simulink library "StdAnimationLibrary2017"  (R2020a)
settings: Solver=VariableStepAuto  StartTime=0.0  StopTime=10.0  RelTol=1e-3
undefined symbols (not defined in the file): CONST_No_Animation, P_AnimationPeriod, P_CIE_GAMMA, P_CIE_PWM, P_DefaultValue, P_EndValue, P_Nb_Seq_Max, P_SequenceNum_perAnim, P_StartValue, P_TRamp, P_TStart
libraries: simulink x5, $bdroot x1
settings Model: Creator=mchawa  LastModifiedBy=oashraf
settings DataIOCC: ReturnWorkspaceOutputs=off
settings DebuggingCC: ArithmeticOperatorsInVariantConditions=warning
settings SFSimCC: SimUseLocalCustomCode=off  CustomCodeUndefinedFunction=UseInterfaceOnly
settings RTWCC: RTWUseLocalCustomCode=off

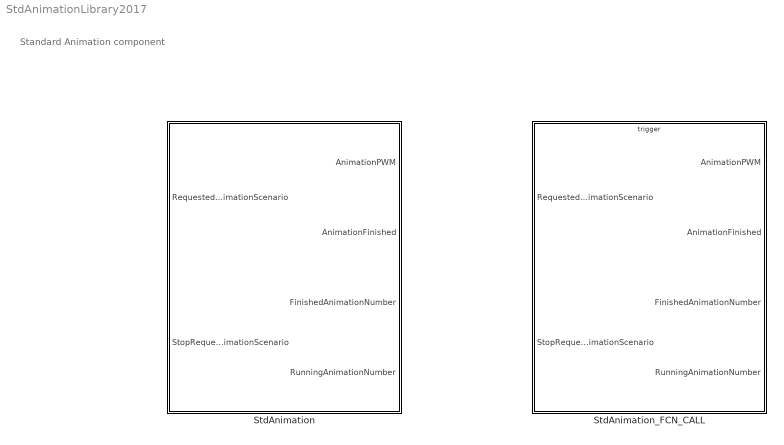
== system StdAnimationLibrary2017 ==
  note: Standard Animation component
  StdAnimation : Subsystem
  StdAnimation_FCN_CALL : Subsystem  TreatAsAtomicUnit=on

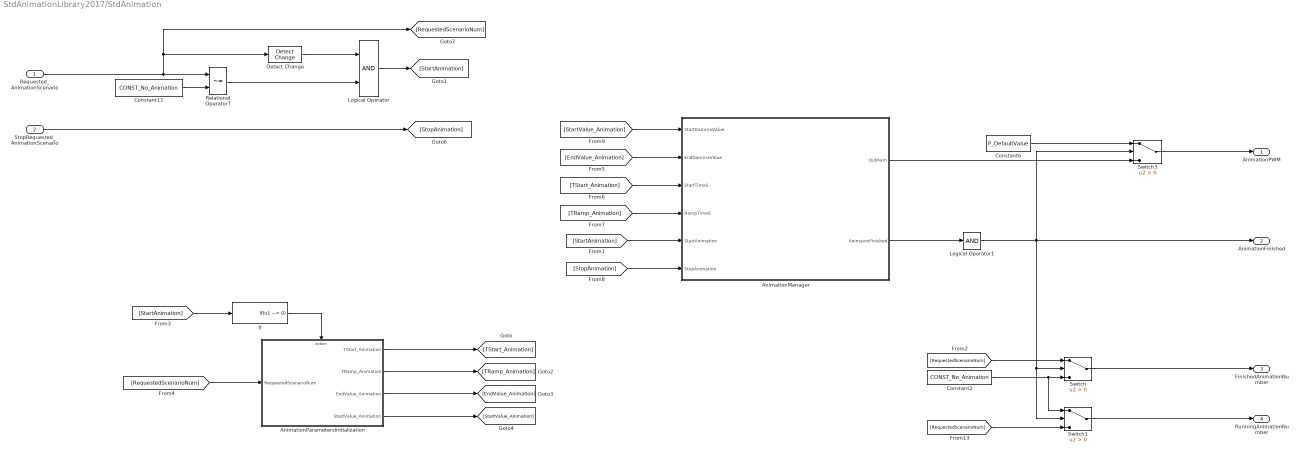
== system StdAnimationLibrary2017/StdAnimation ==
  Requested_AnimationScenario : Inport
  StopRequested_AnimationScenario : Inport  Port=2  PortDimensions=1
  AnimationManager : Subsystem  TreatAsAtomicUnit=on
  AnimationParametersInitialization : Subsystem  TreatAsAtomicUnit=on
  Constant11 : Constant  Value=CONST_No_Animation  OutDataTypeStr=uint8
  Constant2 : Constant  Value=CONST_No_Animation
  Constant6 : Constant  Value=P_DefaultValue
  Detect Change : simulink/Logic and Bit Operations/Detect Change  vinit=0  OutDataTypeStr=boolean
  If : If  IfExpression=u1 ~= 0  ShowElse=off
  Logical Operator : Logic  IconShape=distinctive  AllPortsSameDT=off  OutDataTypeStr=boolean
  Logical Operator1 : Logic  Inputs=1  AllPortsSameDT=off  OutDataTypeStr=boolean
  Relational Operator7 : RelationalOperator  Operator=~=  OutDataTypeStr=boolean  RndMeth=Simplest
  Switch : Switch  Criteria=u2 > Threshold
  Switch1 : Switch  Criteria=u2 > Threshold
  Switch3 : Switch  Criteria=u2 > Threshold
  AnimationPWM : Outport  VectorParamsAs1DForOutWhenUnconnected=off
  AnimationFinished : Outport  Port=2  VectorParamsAs1DForOutWhenUnconnected=off
  FinishedAnimationNumber : Outport  Port=3  VectorParamsAs1DForOutWhenUnconnected=off
  RunningAnimationNumber : Outport  Port=4  VectorParamsAs1DForOutWhenUnconnected=off
  wires:
  AnimationManager/2(AnimaionFinished) -> Logical Operator1/1
  Detect Change/1 -> Logical Operator/1
  AnimationManager/1(OutPwm) -> Switch3/3
  Requested_AnimationScenario/1 -> [RequestedScenarioNum], Detect Change/1, Relational Operator7/1
  [StartAnimation] -> AnimationManager/5(StartAnimation)
  [RequestedScenarioNum] -> Switch1/3
  Logical Operator/1 -> [StartAnimation]
  If/1 -> AnimationParametersInitialization/Action
  [EndValue_Animation] -> AnimationManager/2(EndGammaValue)
  [StartAnimation] -> If/1
  Constant2/1 -> Switch1/1, Switch/3
  [StartValue_Animation] -> AnimationManager/1(StartGammaValue)
  AnimationParametersInitialization/2(TRamp_Animation) -> [TRamp_Animation]
  AnimationParametersInitialization/3(EndValue_Animation) -> [EndValue_Animation]
  [RequestedScenarioNum] -> Switch/1
  Relational Operator7/1 -> Logical Operator/2
  [TStart_Animation] -> AnimationManager/3(StartTimeS)
  [StopAnimation] -> AnimationManager/6(StopAnimation)
  AnimationParametersInitialization/1(TStart_Animation) -> [TStart_Animation]
  [TRamp_Animation] -> AnimationManager/4(RampTimeS)
  Switch1/1 -> RunningAnimationNumber/1
  Switch/1 -> FinishedAnimationNumber/1
  Constant11/1 -> Relational Operator7/2
  StopRequested_AnimationScenario/1 -> [StopAnimation]
  [RequestedScenarioNum] -> AnimationParametersInitialization/1(RequestedScenarioNum)
  Constant6/1 -> Switch3/1
  Switch3/1 -> AnimationPWM/1
  Logical Operator1/1 -> AnimationFinished/1, Switch3/2, Switch/2, Switch1/2
  AnimationParametersInitialization/4(StartValue_Animation) -> [StartValue_Animation]

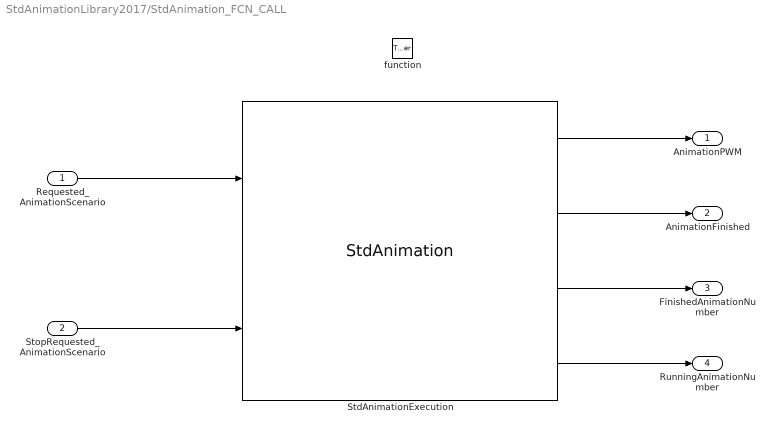
== system StdAnimationLibrary2017/StdAnimation_FCN_CALL ==
  Requested_AnimationScenario : Inport
  StopRequested_AnimationScenario : Inport  Port=2  PortDimensions=1
  function : TriggerPort  TriggerType=function-call  VariantControl=Variant
  StdAnimationExecution : $bdroot/StdAnimation  SystemSampleTime=-1  Latency=0  AutoFrameSizeCalculation=off
      link override AnimationManager/AnimationParametersManager/Detect Change: vinit=P_SequenceNum_perAnim
  AnimationPWM : Outport  VectorParamsAs1DForOutWhenUnconnected=off
  AnimationFinished : Outport  Port=2  VectorParamsAs1DForOutWhenUnconnected=off
  FinishedAnimationNumber : Outport  Port=3  VectorParamsAs1DForOutWhenUnconnected=off
  RunningAnimationNumber : Outport  Port=4  VectorParamsAs1DForOutWhenUnconnected=off
  wires:
  Requested_AnimationScenario/1 -> StdAnimationExecution/1
  StopRequested_AnimationScenario/1 -> StdAnimationExecution/2
  StdAnimationExecution/4 -> RunningAnimationNumber/1
  StdAnimationExecution/3 -> FinishedAnimationNumber/1
  StdAnimationExecution/1 -> AnimationPWM/1
  StdAnimationExecution/2 -> AnimationFinished/1

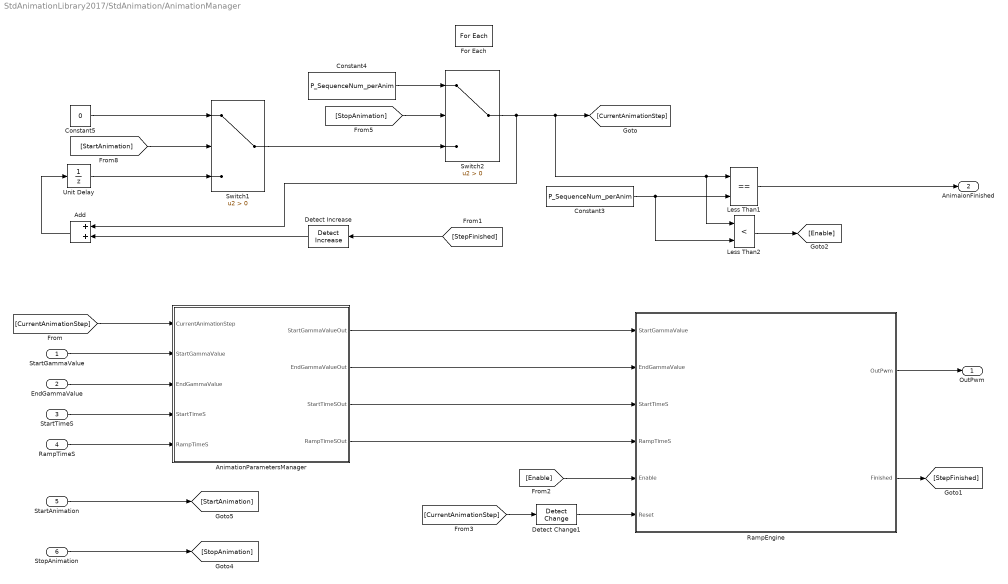
== system StdAnimationLibrary2017/StdAnimation/AnimationManager ==
  StartGammaValue : Inport  Partition=on  PartitionDimension=2  PartitionWidth=1  PartitionOffset=0
  EndGammaValue : Inport  Port=2  Partition=on  PartitionDimension=2  PartitionWidth=1  PartitionOffset=0
  StartTimeS : Inport  Port=3  Partition=on  PartitionDimension=2  PartitionWidth=1  PartitionOffset=0
  RampTimeS : Inport  Port=4  Partition=on  PartitionDimension=2  PartitionWidth=1  PartitionOffset=0
  StartAnimation : Inport  Port=5  OutDataTypeStr=boolean
  StopAnimation : Inport  Port=6  OutDataTypeStr=boolean
  Add : Sum
  AnimationParametersManager : Subsystem  TreatAsAtomicUnit=on
  Constant3 : Constant  Value=P_SequenceNum_perAnim
  Constant4 : Constant  Value=P_SequenceNum_perAnim  OutDataTypeStr=uint8
  Constant5 : Constant  Value=0  OutDataTypeStr=uint8
  Detect Change1 : simulink/Logic and Bit Operations/Detect Change  vinit=0  OutDataTypeStr=boolean
  Detect Increase : simulink/Logic and Bit Operations/Detect Increase  vinit=0.0  OutDataTypeStr=boolean
  For Each : ForEach  DisableCoverage=on
  Less Than1 : RelationalOperator  Operator===  OutDataTypeStr=boolean  RndMeth=Simplest
  Less Than2 : RelationalOperator  Operator=<  OutDataTypeStr=boolean  RndMeth=Simplest
  RampEngine : Subsystem
  Switch1 : Switch  Criteria=u2 > Threshold  OutDataTypeStr=uint8
  Switch2 : Switch  Criteria=u2 > Threshold  OutDataTypeStr=uint8
  Unit Delay : UnitDelay  InitialCondition=P_SequenceNum_perAnim  SampleTime=-1  HasFrameUpgradeWarning=on
  OutPwm : Outport  ConcatenationDimension=1  VectorParamsAs1DForOutWhenUnconnected=off
  AnimaionFinished : Outport  Port=2  ConcatenationDimension=1  VectorParamsAs1DForOutWhenUnconnected=off
  wires:
  [CurrentAnimationStep] -> AnimationParametersManager/1(CurrentAnimationStep)
  Switch1/1 -> Switch2/3
  [CurrentAnimationStep] -> Detect Change1/1
  Constant5/1 -> Switch1/1
  [StartAnimation] -> Switch1/2
  EndGammaValue/1 -> AnimationParametersManager/3(EndGammaValue)
  Unit Delay/1 -> Switch1/3
  Add/1 -> Unit Delay/1
  [Enable] -> RampEngine/5(Enable)
  [StepFinished] -> Detect Increase/1
  Detect Increase/1 -> Add/2
  Constant4/1 -> Switch2/1
  RampEngine/2(Finished) -> [StepFinished]
  [StopAnimation] -> Switch2/2
  AnimationParametersManager/1(StartGammaValueOut) -> RampEngine/1(StartGammaValue)
  AnimationParametersManager/2(EndGammaValueOut) -> RampEngine/2(EndGammaValue)
  StartTimeS/1 -> AnimationParametersManager/4(StartTimeS)
  RampTimeS/1 -> AnimationParametersManager/5(RampTimeS)
  AnimationParametersManager/3(StartTimeSOut) -> RampEngine/3(StartTimeS)
  AnimationParametersManager/4(RampTimeSOut) -> RampEngine/4(RampTimeS)
  StartAnimation/1 -> [StartAnimation]
  StopAnimation/1 -> [StopAnimation]
  Detect Change1/1 -> RampEngine/6(Reset)
  RampEngine/1(OutPwm) -> OutPwm/1
  Constant3/1 -> Less Than1/2, Less Than2/2
  StartGammaValue/1 -> AnimationParametersManager/2(StartGammaValue)
  Switch2/1 -> Less Than2/1, Less Than1/1, [CurrentAnimationStep], Add/1
  Less Than1/1 -> AnimaionFinished/1
  Less Than2/1 -> [Enable]

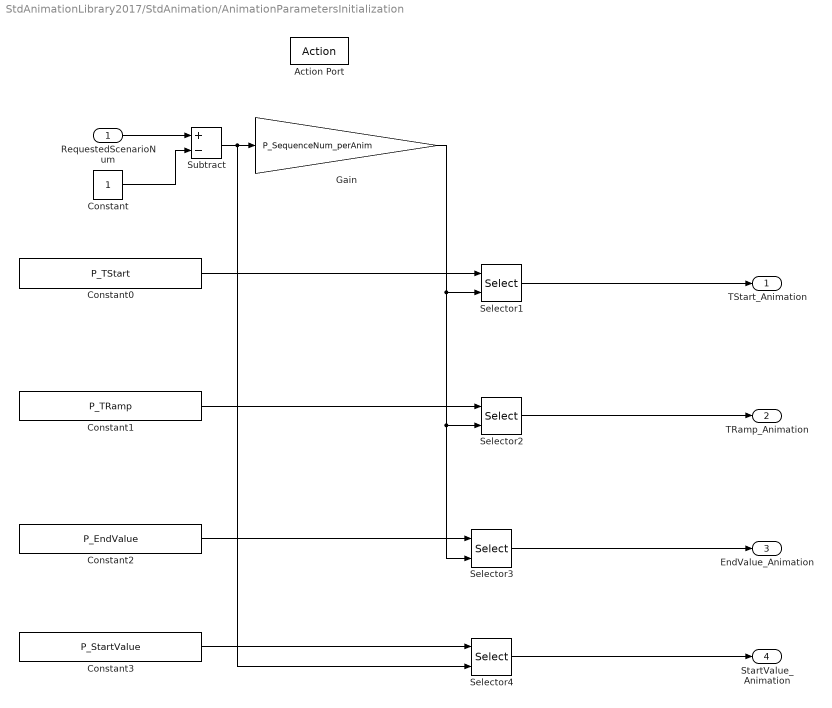
== system StdAnimationLibrary2017/StdAnimation/AnimationParametersInitialization ==
  RequestedScenarioNum : Inport
  Action Port : ActionPort  ActionPortLabel=if { }
  Constant : Constant  OutDataTypeStr=uint8
  Constant0 : Constant  Value=P_TStart
  Constant1 : Constant  Value=P_TRamp
  Constant2 : Constant  Value=P_EndValue
  Constant3 : Constant  Value=P_StartValue
  Gain : Gain  Gain=P_SequenceNum_perAnim  OutDataTypeStr=uint8
  Selector1 : Selector  NumberOfDimensions=2  IndexMode=Zero-based  InputPortWidth=3  IndexOptions=Starting index (port),Select all  Indices=[1 3],1  OutputSizes=P_SequenceNum_perAnim,1
  Selector2 : Selector  NumberOfDimensions=2  IndexMode=Zero-based  InputPortWidth=3  IndexOptions=Starting index (port),Select all  Indices=[1 3],1  OutputSizes=P_SequenceNum_perAnim,1
  Selector3 : Selector  NumberOfDimensions=2  IndexMode=Zero-based  InputPortWidth=3  IndexOptions=Starting index (port),Select all  Indices=[1 3],1  OutputSizes=P_SequenceNum_perAnim,1
  Selector4 : Selector  NumberOfDimensions=2  IndexMode=Zero-based  InputPortWidth=3  IndexOptions=Index vector (port),Select all  Indices=[1 3],1  OutputSizes=P_Nb_Seq_Max,1
  Subtract : Sum  Inputs=+-
  TStart_Animation : Outport  VectorParamsAs1DForOutWhenUnconnected=off
  TRamp_Animation : Outport  Port=2  VectorParamsAs1DForOutWhenUnconnected=off
  EndValue_Animation : Outport  Port=3  VectorParamsAs1DForOutWhenUnconnected=off
  StartValue_Animation : Outport  Port=4  VectorParamsAs1DForOutWhenUnconnected=off
  wires:
  Constant0/1 -> Selector1/1
  Selector1/1 -> TStart_Animation/1
  Selector2/1 -> TRamp_Animation/1
  Selector3/1 -> EndValue_Animation/1
  Constant2/1 -> Selector3/1
  Constant1/1 -> Selector2/1
  Gain/1 -> Selector3/2, Selector2/2, Selector1/2
  Subtract/1 -> Selector4/2, Gain/1
  RequestedScenarioNum/1 -> Subtract/1
  Constant/1 -> Subtract/2
  Constant3/1 -> Selector4/1
  Selector4/1 -> StartValue_Animation/1

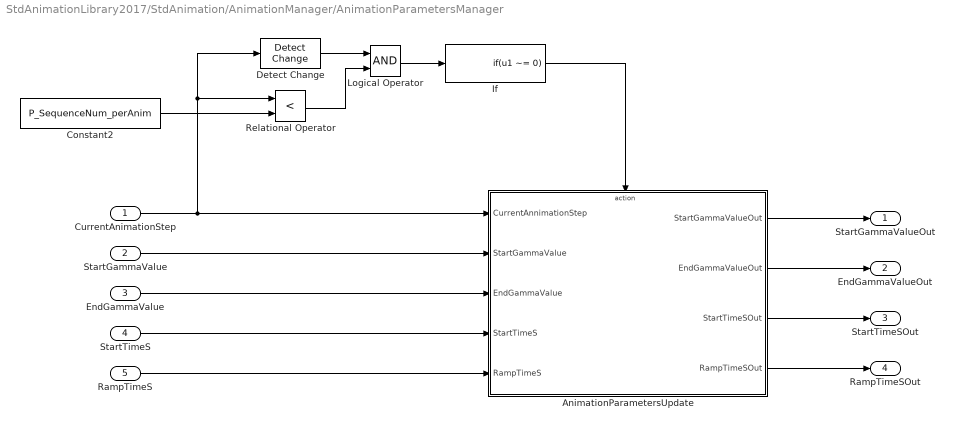
== system StdAnimationLibrary2017/StdAnimation/AnimationManager/AnimationParametersManager ==
  CurrentAnimationStep : Inport  OutDataTypeStr=uint8
  StartGammaValue : Inport  Port=2  OutDataTypeStr=uint8
  EndGammaValue : Inport  Port=3
  StartTimeS : Inport  Port=4
  RampTimeS : Inport  Port=5
  AnimationParametersUpdate : Subsystem  TreatAsAtomicUnit=on
  Constant2 : Constant  Value=P_SequenceNum_perAnim
  Detect Change : simulink/Logic and Bit Operations/Detect Change  vinit=0  OutDataTypeStr=boolean
  If : If  IfExpression=u1 ~= 0  ShowElse=off
  Logical Operator : Logic  AllPortsSameDT=off  OutDataTypeStr=boolean
  Relational Operator : RelationalOperator  Operator=<  OutDataTypeStr=boolean  RndMeth=Simplest
  StartGammaValueOut : Outport  VectorParamsAs1DForOutWhenUnconnected=off
  EndGammaValueOut : Outport  Port=2  VectorParamsAs1DForOutWhenUnconnected=off
  StartTimeSOut : Outport  Port=3  VectorParamsAs1DForOutWhenUnconnected=off
  RampTimeSOut : Outport  Port=4  VectorParamsAs1DForOutWhenUnconnected=off
  wires:
  EndGammaValue/1 -> AnimationParametersUpdate/3(EndGammaValue)
  CurrentAnimationStep/1 -> AnimationParametersUpdate/1(CurrentAnnimationStep), Relational Operator/1, Detect Change/1
  If/1 -> AnimationParametersUpdate/Action
  Logical Operator/1 -> If/1
  Detect Change/1 -> Logical Operator/1
  Relational Operator/1 -> Logical Operator/2
  StartTimeS/1 -> AnimationParametersUpdate/4(StartTimeS)
  RampTimeS/1 -> AnimationParametersUpdate/5(RampTimeS)
  AnimationParametersUpdate/1(StartGammaValueOut) -> StartGammaValueOut/1
  AnimationParametersUpdate/2(EndGammaValueOut) -> EndGammaValueOut/1
  AnimationParametersUpdate/3(StartTimeSOut) -> StartTimeSOut/1
  AnimationParametersUpdate/4(RampTimeSOut) -> RampTimeSOut/1
  Constant2/1 -> Relational Operator/2
  StartGammaValue/1 -> AnimationParametersUpdate/2(StartGammaValue)

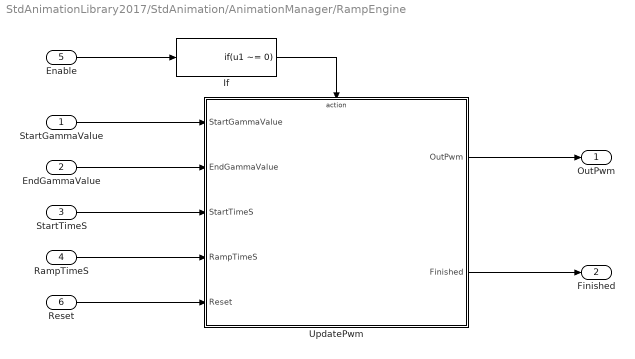
== system StdAnimationLibrary2017/StdAnimation/AnimationManager/RampEngine ==
  StartGammaValue : Inport
  EndGammaValue : Inport  Port=2
  StartTimeS : Inport  Port=3
  RampTimeS : Inport  Port=4
  Enable : Inport  Port=5
  Reset : Inport  Port=6  OutDataTypeStr=boolean
  If : If  IfExpression=u1 ~= 0  ShowElse=off
  UpdatePwm : Subsystem  TreatAsAtomicUnit=on
  OutPwm : Outport  VectorParamsAs1DForOutWhenUnconnected=off
  Finished : Outport  Port=2  VectorParamsAs1DForOutWhenUnconnected=off
  wires:
  If/1 -> UpdatePwm/Action
  Enable/1 -> If/1
  StartGammaValue/1 -> UpdatePwm/1(StartGammaValue)
  EndGammaValue/1 -> UpdatePwm/2(EndGammaValue)
  StartTimeS/1 -> UpdatePwm/3(StartTimeS)
  RampTimeS/1 -> UpdatePwm/4(RampTimeS)
  Reset/1 -> UpdatePwm/5(Reset)
  UpdatePwm/1(OutPwm) -> OutPwm/1
  UpdatePwm/2(Finished) -> Finished/1

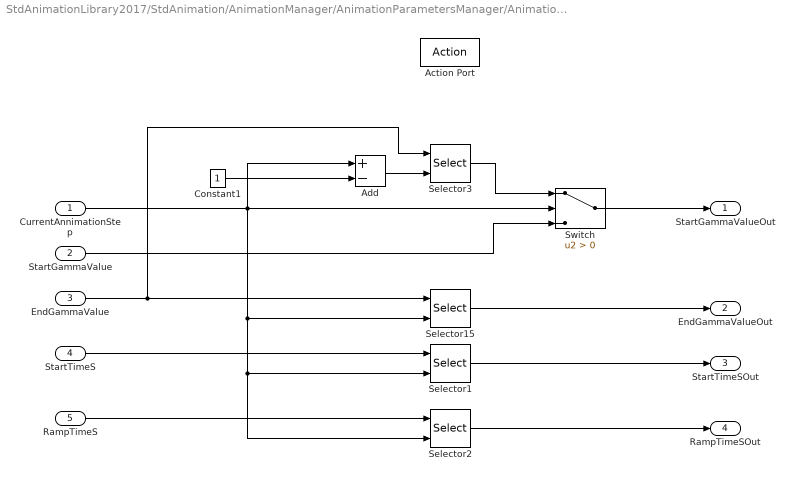
== system StdAnimationLibrary2017/StdAnimation/AnimationManager/AnimationParametersManager/AnimationParametersUpdate ==
  CurrentAnnimationStep : Inport  OutDataTypeStr=uint8
  StartGammaValue : Inport  Port=2
  EndGammaValue : Inport  Port=3
  StartTimeS : Inport  Port=4
  RampTimeS : Inport  Port=5
  Action Port : ActionPort
  Add : Sum  Inputs=+-
  Constant1 : Constant  OutDataTypeStr=uint8
  Selector{1..3,15} (4 alike) : Selector  IndexMode=Zero-based  InputPortWidth=P_SequenceNum_perAnim  IndexOptions=Index vector (port)  Indices=[1 3]  OutputSizes=1
  Switch : Switch  Criteria=u2 > Threshold
  StartGammaValueOut : Outport  VectorParamsAs1DForOutWhenUnconnected=off
  EndGammaValueOut : Outport  Port=2  VectorParamsAs1DForOutWhenUnconnected=off
  StartTimeSOut : Outport  Port=3  VectorParamsAs1DForOutWhenUnconnected=off
  RampTimeSOut : Outport  Port=4  VectorParamsAs1DForOutWhenUnconnected=off
  wires:
  Selector1/1 -> StartTimeSOut/1
  Selector15/1 -> EndGammaValueOut/1
  EndGammaValue/1 -> Selector15/1, Selector3/1
  Selector2/1 -> RampTimeSOut/1
  StartGammaValue/1 -> Switch/3
  Selector3/1 -> Switch/1
  Add/1 -> Selector3/2
  StartTimeS/1 -> Selector1/1
  RampTimeS/1 -> Selector2/1
  CurrentAnnimationStep/1 -> Selector15/2, Selector1/2, Selector2/2, Add/1, Switch/2
  Switch/1 -> StartGammaValueOut/1
  Constant1/1 -> Add/2

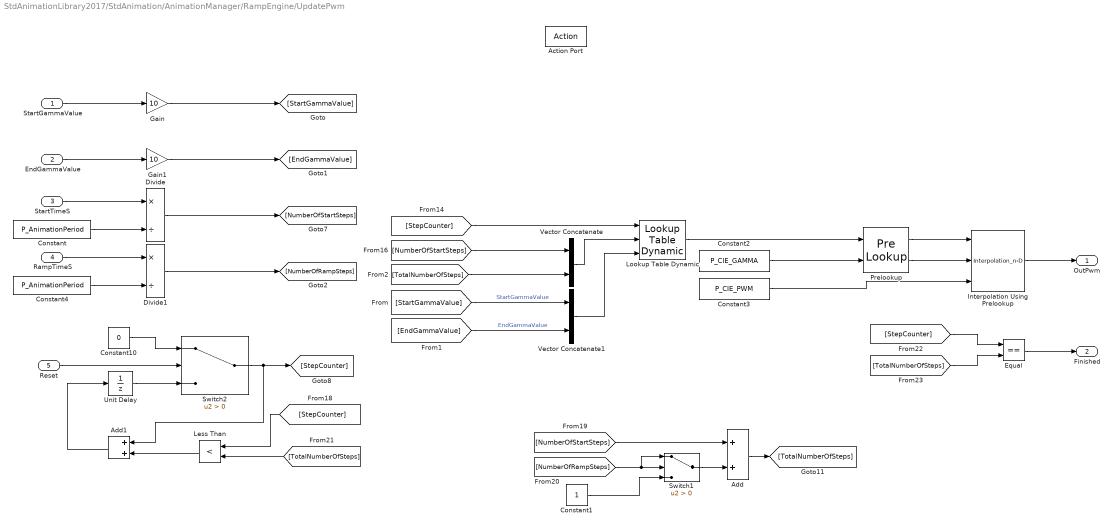
== system StdAnimationLibrary2017/StdAnimation/AnimationManager/RampEngine/UpdatePwm ==
  StartGammaValue : Inport
  EndGammaValue : Inport  Port=2
  StartTimeS : Inport  Port=3
  RampTimeS : Inport  Port=4
  Reset : Inport  Port=5  OutDataTypeStr=boolean
  Action Port : ActionPort
  Add : Sum
  Add1 : Sum
  Constant : Constant  Value=P_AnimationPeriod
  Constant1 : Constant  OutDataTypeStr=uint16
  Constant10 : Constant  Value=0  OutDataTypeStr=uint8
  Constant2 : Constant  Value=P_CIE_GAMMA
  Constant3 : Constant  Value=P_CIE_PWM
  Constant4 : Constant  Value=P_AnimationPeriod
  Divide : Product  Inputs=*/  OutDataTypeStr=uint16
  Divide1 : Product  Inputs=*/  OutDataTypeStr=uint16
  Equal : RelationalOperator  Operator===  OutDataTypeStr=boolean  RndMeth=Simplest
  Gain : Gain  Gain=10  OutDataTypeStr=uint16
  Gain1 : Gain  Gain=10  OutDataTypeStr=uint16
  Interpolation Using Prelookup : Interpolation_n-D  NumberOfTableDimensions=1  TableSource=Input port  ExtrapMethod=Clip  RemoveProtectionIndex=on  ValidIndexMayReachLast=on  InternalRulePriority=Speed
      settings: InputPortMap=u0,u1,p2
  Less Than : RelationalOperator  Operator=<  OutDataTypeStr=boolean  RndMeth=Simplest
  Lookup Table Dynamic : simulink/Lookup Tables/Lookup Table Dynamic  LookUpMeth=Interpolation-Use End Values  OutDataType=fixdt('uint16')  OutScaling=[]  OutputDataTypeScalingMode=Specify via dialog  OutDataTypeStr=uint16  DoSatur=off
  Prelookup : PreLookup  BreakpointsDataSource=Input port  BreakpointsData=[10:10:110]  BreakpointObject=P_CIE_GAMMA  IndexSearchMethod=Linear search  UseLastBreakpoint=on  RemoveProtectionInput=on  IndexDataTypeStr=uint16
      settings: InputPortMap=u0,p1
  Switch1 : Switch  Criteria=u2 > Threshold
  Switch2 : Switch  Criteria=u2 > Threshold  OutDataTypeStr=uint16
  Unit Delay : UnitDelay  SampleTime=-1  HasFrameUpgradeWarning=on
  Vector Concatenate : Concatenate
  Vector Concatenate1 : Concatenate
  OutPwm : Outport  VectorParamsAs1DForOutWhenUnconnected=off
  Finished : Outport  Port=2  VectorParamsAs1DForOutWhenUnconnected=off
  wires:
  [StepCounter] -> Less Than/1
  Divide/1 -> [NumberOfStartSteps]
  [NumberOfStartSteps] -> Vector Concatenate/1
  Reset/1 -> Switch2/2
  RampTimeS/1 -> Divide1/1
  StartTimeS/1 -> Divide/1
  Unit Delay/1 -> Switch2/3
  Constant10/1 -> Switch2/1
  Add1/1 -> Unit Delay/1
  [TotalNumberOfSteps] -> Equal/2
  StartGammaValue/1 -> Gain/1
  Divide1/1 -> [NumberOfRampSteps]
  Equal/1 -> Finished/1
  [StepCounter] -> Equal/1
  EndGammaValue/1 -> Gain1/1
  [TotalNumberOfSteps] -> Less Than/2
  Less Than/1 -> Add1/2
  Switch2/1 -> [StepCounter], Add1/1
  Vector Concatenate1/1 -> Lookup Table Dynamic/3
  Vector Concatenate/1 -> Lookup Table Dynamic/2
  [StepCounter] -> Lookup Table Dynamic/1
  [TotalNumberOfSteps] -> Vector Concatenate/2
  [StartGammaValue] -> Vector Concatenate1/1  "StartGammaValue"
  [EndGammaValue] -> Vector Concatenate1/2  "EndGammaValue"
  Constant2/1 -> Prelookup/2
  Lookup Table Dynamic/1 -> Prelookup/1
  Prelookup/2 -> Interpolation Using Prelookup/2
  Prelookup/1 -> Interpolation Using Prelookup/1
  Constant3/1 -> Interpolation Using Prelookup/3
  Interpolation Using Prelookup/1 -> OutPwm/1
  Gain/1 -> [StartGammaValue]
  Gain1/1 -> [EndGammaValue]
  Constant1/1 -> Switch1/3
  [NumberOfRampSteps] -> Switch1/2, Switch1/1
  [NumberOfStartSteps] -> Add/1
  Switch1/1 -> Add/2
  Add/1 -> [TotalNumberOfSteps]
  Constant/1 -> Divide/2
  Constant4/1 -> Divide1/2
